simulink model "Simulator"  (R2015a)
settings: Solver=ode45  StartTime=0.0  StopTime=tsim  RelTol=1e-3
InitFcn:
  | Parameters
values from neighbouring files (symbols this model uses):
  delay_altitude = 1    [Parameters_controllers.m]
  delay_attitude = 1    [Parameters_controllers.m]
  delay_mixer = 1    [Parameters_controllers.m]
  dLMN = [dLdp  0   0 ... (first row only)    [Parameters.m]    (also in Parameters_quadrotor.m = [dL_dp  0    0)
  g = 9.81    [Parameters.m]
  In = diag([Ixx Iyy Izz])    [Parameters.m]
  InInv = In\eye(3)    [Parameters.m]
  K = param*sign    [Parameters.m]    (also in Parameters_controllers.m = [              -Kt,               -Kt,               -Kt,   )
  Kdp = 0.05    [Parameters.m]
  Kdq = 0.05    [Parameters.m]
  Kinv = K\eye(4)    [Parameters.m]    (also in Parameters_controllers.m = [ -1/(4*Kt),  2^(1/2)/(4*Kt*b),  2^(1/2)/(4*Kt*b), -1/(4*Kq))
  Kip = 0.3    [Parameters.m]
  Kiq = 0.3    [Parameters.m]
  Kir = 0.01    [Parameters.m]
  KPP = 1.1    [Parameters.m]
  Kpp = 0.3    [Parameters.m]
  Kpq = 0.3    [Parameters.m]
  Kpr = 0.08    [Parameters.m]
  KRP = 1.1    [Parameters.m]
  m = 1.5    [Parameters.m]
  Mb = diag([m m m])    [Parameters.m]
  MbInv = Mb\eye(3)    [Parameters.m]
  N = 1/Tf    (= 100)    [Parameters.m]
  pitchMax = pi/6    (= 0.523598775598)    [Parameters.m]
  rollMax = pi/6    (= 0.523598775598)    [Parameters.m]
  tau = 0.055257    [Parameters.m]
  x1 = [m q]    [Parameters.m]
undefined symbols (not defined in the file or in its folder): KaD, KaI, KaN, KaP, Kba, Kbp, Kbq, Kbr, KD, Kdr, KN, KP, KPD, KPI, KRD, KRI, KYD, KYP, magnitude, sat, sata, satp, satq, satr, sigbuilder_block, tc, U
libraries: simulink x9, aerolibutil x2
settings Model: Creator=pela  LastModifiedBy=Mattia
settings SolverCC: ZeroCrossAlgorithm=Adaptive
settings DataIOCC: LimitDataPoints=off

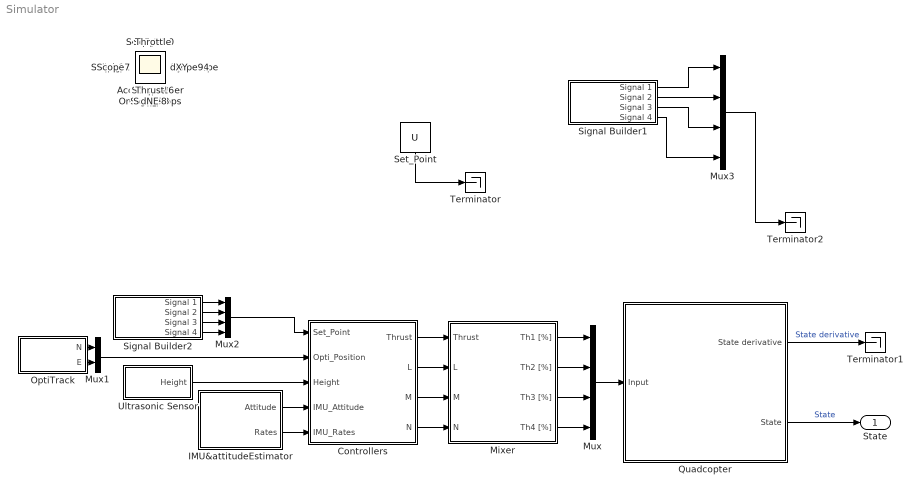
== system Simulator ==
  Controllers : Subsystem
  IMU&attitudeEstimator : Subsystem
  Mixer : Subsystem  InitFcn=|
      | %%Parameters definition
      | b = 0.55/2;
      | RPMmax = 3*4.2*710;
      | D = 12*2.54/100;
      | Ct = 0.001;
      | Cq = 0.001;
      | ro = 1.225;
      | 
      | %% From omega squared to forces/torques
      |  A = ro*D^4*diag([Ct b/sqrt(2)*Ct b/sqrt(2)*Ct Cq*D]);
      |  B = [ 1  1  1 1;
      |          1 -1 -1 1;
      |         -1 -1  1 1;
      |         -1  1 -1 1];
      |  C = inv(A*B);       %TM = C * omegasq
  Mux : Mux
  Mux1 : Mux  Inputs=2
  Mux2 : Mux
  Mux3 : Mux
  OptiTrack : Subsystem
  Quadcopter : Subsystem
      mask Display:
      | image(imread('quad.png'))
      | port_label('input',1,'u')
      | port_label('output',1,'Xdot')
      | port_label('output',2,'X')
  Set_Point : Constant  Value=U
  Signal Builder1 : Subsystem  Tag=STV Subsys  LoadFcn=sigbuilder_block('load');  StartFcn=sigbuilder_block('start');  StopFcn=sigbuilder_block('stop');  ClipboardFcn=sigbuilder_block('clipboard');  mask(Sigbuilder block){}
      mask help: Simulink:masks:SigbuilderBlock_MD
      mask init:
      | if ~strcmp(get_param(bdroot(gcbh),'SimulationStatus'),'stopped') tuvar = sigbuilder_block('maskInit'); end
      settings: CopyFcn=sigbuilder_block('copy');  DeleteFcn=sigbuilder_block('delete');  ModelCloseFcn=sigbuilder_block('modelClose');  PreSaveFcn=sigbuilder_block('preSave');  PauseFcn=sigbuilder_block('pause');  ContinueFcn=sigbuilder_block('continue');  NameChangeFcn=sigbuilder_block('namechange');  OpenFcn=sigbuilder_block('open',[5.4 30 1141.2 522.6 ]);  CloseFcn=sigbuilder_block('close');
      mask Display: plot(0, 0, 100, 100,[2, 2, 32, 32, 2], [68, 8, 8, 68, 68],[32, 2], [38, 38], [32, 19, 2],[53, 60, 44], [32, 17, 17, 2],[16, 16, 31, 31]);txt = getActiveGroup(gcbh);text(2, 100, txt,'verticalAlignment', 'top');
  Signal Builder2 : Subsystem  Tag=STV Subsys  LoadFcn=sigbuilder_block('load');  StartFcn=sigbuilder_block('start');  StopFcn=sigbuilder_block('stop');  ClipboardFcn=sigbuilder_block('clipboard');  mask(Sigbuilder block){}
      mask help: Simulink:masks:SigbuilderBlock_MD
      mask init:
      | if ~strcmp(get_param(bdroot(gcbh),'SimulationStatus'),'stopped') tuvar = sigbuilder_block('maskInit'); end
      settings: CopyFcn=sigbuilder_block('copy');  DeleteFcn=sigbuilder_block('delete');  ModelCloseFcn=sigbuilder_block('modelClose');  PreSaveFcn=sigbuilder_block('preSave');  PauseFcn=sigbuilder_block('pause');  ContinueFcn=sigbuilder_block('continue');  NameChangeFcn=sigbuilder_block('namechange');  OpenFcn=sigbuilder_block('open',[5.4 30 1141.2 522.6 ]);  CloseFcn=sigbuilder_block('close');
      mask Display: plot(0, 0, 100, 100,[2, 2, 32, 32, 2], [68, 8, 8, 68, 68],[32, 2], [38, 38], [32, 19, 2],[53, 60, 44], [32, 17, 17, 2],[16, 16, 31, 31]);txt = getActiveGroup(gcbh);text(2, 100, txt,'verticalAlignment', 'top');
  Terminator : Terminator
  Terminator1 : Terminator
  Terminator2 : Terminator
  Ultrasonic Sensor : Subsystem
  State : Outport
  Accelerometer : Scope
      settings: ShowLegends=on  YMin=-10  YMax=10  SaveName=ScopeData9
  Fg : Scope
      settings: ShowLegends=on  YMin=-10  YMax=10  SaveName=ScopeData4
  Fprops : Scope
      settings: ShowLegends=on  YMin=-22.13861  YMax=2.45985  SaveName=ScopeData2
  Gyroscope : Scope
      settings: ShowLegends=on  YMin=-10  YMax=10  SaveName=ScopeData10
  Height : Scope
      settings: ShowLegends=on  TimeRange=10  YMin=-0.2  YMax=1.4  SaveName=ScopeData5
  Moments : Scope
      settings: YMin=-1.875  YMax=1.875  SaveName=ScopeData7
  Mprops : Scope
      settings: ShowLegends=on  YMin=-0.25293  YMax=0.32754  SaveName=ScopeData3
  Omega_props : Scope
      settings: ShowLegends=on  TimeRange=10  YMin=328.24586  YMax=550.97691
  Scope{,1..16} (17 alike) : Scope
      Scope settings: YMin=-1.28463  YMax=0.42301  SaveName=ScopeData8
      Scope1 settings: YMin=-10  YMax=10  SaveName=ScopeData11
      Scope10 settings: YMin=-10  YMax=10  SaveName=ScopeData17
      Scope11 settings: YMin=-10  YMax=10  SaveName=ScopeData18
      Scope12 settings: YMin=103280.52588  YMax=299110.73241  SaveName=ScopeData19
      Scope13 settings: YMin=-10  YMax=10  SaveName=ScopeData23
      Scope14 settings: YMin=-10  YMax=10  SaveName=ScopeData26
      Scope15 settings: YMin=-0.00000000000000007  YMax=0.00000000000000005  SaveName=ScopeData27
      Scope16 settings: YMin=-0.07851  YMax=0.5905  SaveName=ScopeData28
      Scope2 settings: YMin=-10  YMax=10  SaveName=ScopeData12
      Scope3 settings: YMin=-10  YMax=10  SaveName=ScopeData13
      Scope4 settings: YMin=-10  YMax=10  SaveName=ScopeData14
      Scope5 settings: YMin=-10  YMax=10  SaveName=ScopeData15
      Scope6 settings: YMin=-10  YMax=10  SaveName=ScopeData20
      Scope7 settings: YMin=-0.0134  YMax=0.02255  SaveName=ScopeData21
      Scope8 settings: YMin=-0.0504  YMax=0.30441  SaveName=ScopeData22
      Scope9 settings: YMin=-10  YMax=10  SaveName=ScopeData16
  Throttle : Scope
      settings: ShowLegends=on  YMin=-12.5  YMax=112.5
  Thrust : Scope
      settings: YMin=-20.52889  YMax=-13.37103  SaveName=ScopeData6
  dNE : Scope
      settings: ShowLegends=on  YMin=-0.125  YMax=1.125  SaveName=ScopeData24
  dXY : Scope
      settings: YMin=-0.125  YMax=1.125  SaveName=ScopeData25
  wires:
  Quadcopter/2(State) -> State/1  "State"
  Mux/1 -> Quadcopter/1(Input)
  Mixer/1(Th1 [%]) -> Mux/1
  Mixer/2(Th2 [%]) -> Mux/2
  Mixer/3(Th3 [%]) -> Mux/3
  Mixer/4(Th4 [%]) -> Mux/4
  Quadcopter/1(State derivative) -> Terminator1/1  "State derivative"
  Ultrasonic Sensor/1(Height) -> Controllers/3(Height)
  Controllers/1(Thrust) -> Mixer/1(Thrust)
  Controllers/2(L) -> Mixer/2(L)
  Controllers/3(M) -> Mixer/3(M)
  Controllers/4(N) -> Mixer/4(N)
  IMU&attitudeEstimator/1(Attitude) -> Controllers/4(IMU_Attitude)
  IMU&attitudeEstimator/2(Rates) -> Controllers/5(IMU_Rates)
  Mux1/1 -> Controllers/2(Opti_Position)
  Mux2/1 -> Controllers/1(Set_Point)
  Set_Point/1 -> Terminator/1
  Signal Builder2/2(Signal 2) -> Mux2/2
  Signal Builder2/3(Signal 3) -> Mux2/3
  Signal Builder2/4(Signal 4) -> Mux2/4
  OptiTrack/1(N) -> Mux1/1
  OptiTrack/2(E) -> Mux1/2
  Signal Builder2/1(Signal 1) -> Mux2/1
  Mux3/1 -> Terminator2/1
  Signal Builder1/2(Signal 2) -> Mux3/2
  Signal Builder1/3(Signal 3) -> Mux3/3
  Signal Builder1/4(Signal 4) -> Mux3/4
  Signal Builder1/1(Signal 1) -> Mux3/1

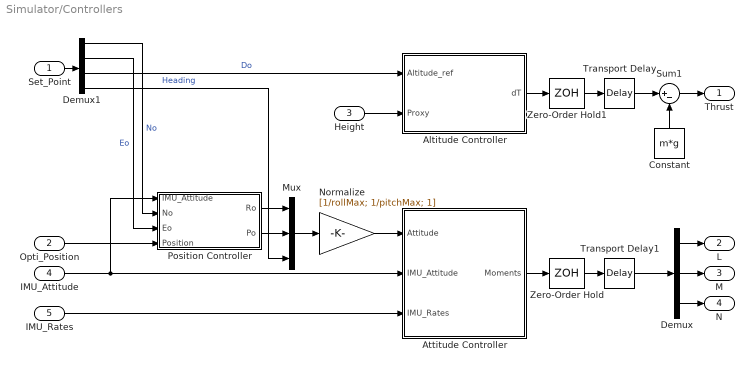
== system Simulator/Controllers ==
  Set_Point : Inport
  Opti_Position : Inport  Port=2
  Height : Inport  Port=3
  IMU_Attitude : Inport  Port=4
  IMU_Rates : Inport  Port=5
  Altitude Controller : Subsystem
  Attitude Controller : Subsystem
  Constant : Constant  Value=m*g
  Demux : Demux  Outputs=3
  Demux1 : Demux
  Mux : Mux  Inputs=3
  Normalize : Gain  Gain=[1/rollMax; 1/pitchMax; 1]
  Position Controller : Subsystem
  Sum1 : Sum  Inputs=|+-
  Transport Delay : TransportDelay  DelayTime=delay_altitude*tc
  Transport Delay1 : TransportDelay  DelayTime=delay_attitude*tc
  Zero-Order Hold : ZeroOrderHold  SampleTime=tc
  Zero-Order Hold1 : ZeroOrderHold  SampleTime=tc
  Thrust : Outport
  L : Outport  Port=2
  M : Outport  Port=3
  N : Outport  Port=4
  wires:
  Attitude Controller/1(Moments) -> Zero-Order Hold/1
  IMU_Rates/1 -> Attitude Controller/3(IMU_Rates)
  Demux/1 -> L/1
  Demux/2 -> M/1
  Demux/3 -> N/1
  Set_Point/1 -> Demux1/1
  IMU_Attitude/1 -> Position Controller/1(IMU_Attitude), Attitude Controller/2(IMU_Attitude)
  Mux/1 -> Normalize/1
  Normalize/1 -> Attitude Controller/1(Attitude)
  Sum1/1 -> Thrust/1
  Height/1 -> Altitude Controller/2(Proxy)
  Altitude Controller/1(dT) -> Zero-Order Hold1/1
  Zero-Order Hold/1 -> Transport Delay1/1
  Zero-Order Hold1/1 -> Transport Delay/1
  Transport Delay1/1 -> Demux/1
  Opti_Position/1 -> Position Controller/4(Position)
  Demux1/1 -> Position Controller/2(No)  "No"
  Demux1/2 -> Position Controller/3(Eo)  "Eo"
  Demux1/3 -> Altitude Controller/1(Altitude_ref)  "Do"
  Demux1/4 -> Mux/3  "Heading"
  Position Controller/1(Ro) -> Mux/1
  Position Controller/2(Po) -> Mux/2
  Transport Delay/1 -> Sum1/1
  Constant/1 -> Sum1/2

== system Simulator/IMU&attitudeEstimator ==
  Zero-Order Hold : ZeroOrderHold  SampleTime=tc
  Zero-Order Hold1 : ZeroOrderHold  SampleTime=tc
  Attitude : Outport
  Rates : Outport  Port=2
  wires:
  [Omega_b] -> Zero-Order Hold1/1
  [Alpha_e] -> Zero-Order Hold/1
  Zero-Order Hold/1 -> Attitude/1
  Zero-Order Hold1/1 -> Rates/1

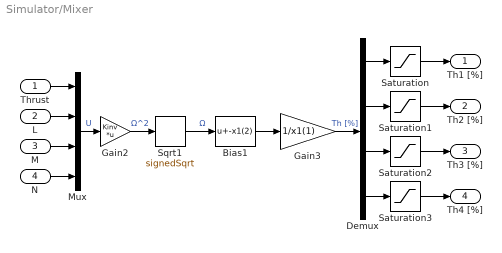
== system Simulator/Mixer ==
  Thrust : Inport
  L : Inport  Port=2
  M : Inport  Port=3
  N : Inport  Port=4
  Bias1 : Bias  Bias=-x1(2)
  Demux : Demux
  Gain2 : Gain  Gain=Kinv  Multiplication=Matrix(K*u)
  Gain3 : Gain  Gain=1/x1(1)
  Mux : Mux
  Saturation{,1..3} (4 alike) : Saturate  UpperLimit=100  LowerLimit=0
  Sqrt1 : Sqrt  Operator=signedSqrt  SaturateOnIntegerOverflow=on
  Th1 [%] : Outport
  Th2 [%] : Outport  Port=2
  Th3 [%] : Outport  Port=3
  Th4 [%] : Outport  Port=4
  wires:
  N/1 -> Mux/4
  M/1 -> Mux/3
  L/1 -> Mux/2
  Demux/1 -> Saturation/1
  Saturation/1 -> Th1 [%]/1
  Demux/2 -> Saturation1/1
  Demux/3 -> Saturation2/1
  Demux/4 -> Saturation3/1
  Saturation3/1 -> Th4 [%]/1
  Saturation2/1 -> Th3 [%]/1
  Saturation1/1 -> Th2 [%]/1
  Gain3/1 -> Demux/1  "Th [%]"
  Bias1/1 -> Gain3/1
  Gain2/1 -> Sqrt1/1  "Ω^2"
  Mux/1 -> Gain2/1  "U"
  Sqrt1/1 -> Bias1/1  "Ω"
  Thrust/1 -> Mux/1

== system Simulator/OptiTrack ==
  Demux : Demux  Outputs=3
  Terminator : Terminator
  N : Outport
  E : Outport  Port=2
  wires:
  Demux/1 -> N/1  "N"
  Demux/3 -> Terminator/1  "D"
  [P_e] -> Demux/1
  Demux/2 -> E/1  "E"

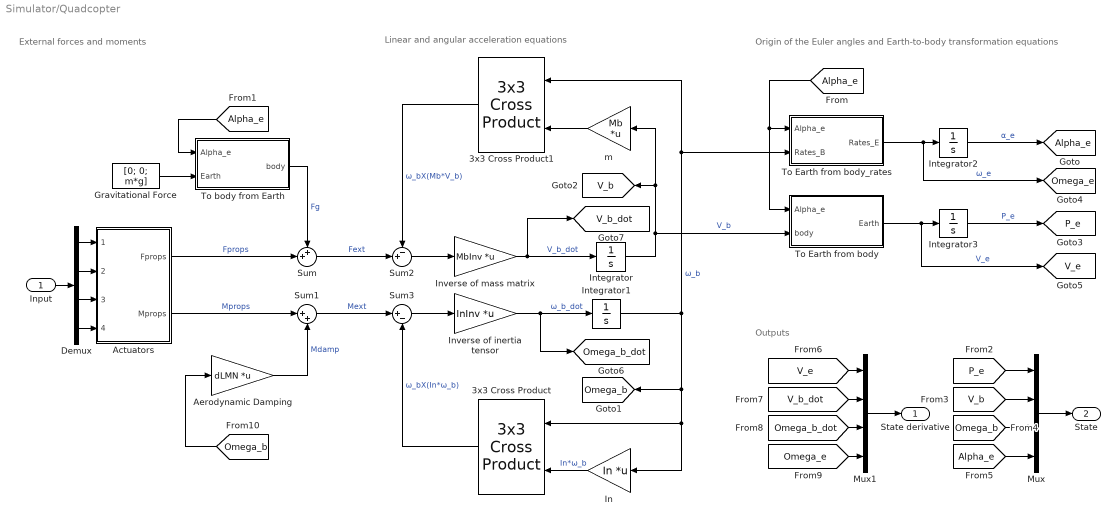
== system Simulator/Quadcopter ==
  note: External forces and moments
  note: Outputs
  note: Origin of the Euler angles and Earth-to-body transformation equations
  note: Linear and angular acceleration equations
  Input : Inport
  3x3 Cross Product : aerolibutil/3x3 Cross Product
  3x3 Cross Product1 : aerolibutil/3x3 Cross Product
  Actuators : Subsystem
  Aerodynamic Damping : Gain  Gain=dLMN  Multiplication=Matrix(K*u)
  Demux : Demux
  Gravitational Force : Constant  Value=[0; 0; m*g]
  In : Gain  Gain=In  Multiplication=Matrix(K*u)
  Integrator{,1..3} (4 alike) : Integrator  InitialCondition=[0; 0; 0]
  Inverse of inertia tensor : Gain  Gain=InInv  Multiplication=Matrix(K*u)
  Inverse of mass matrix : Gain  Gain=MbInv  Multiplication=Matrix(K*u)
  Mux : Mux
  Mux1 : Mux
  Sum : Sum  Inputs=++|
  Sum1 : Sum  Inputs=|++
  Sum2 : Sum  Inputs=-+|
  Sum3 : Sum  Inputs=|+-
  To Earth from body : MATLAB Function  TreatAsAtomicUnit=on
  To Earth from body_rates : MATLAB Function  TreatAsAtomicUnit=on
  To body from Earth : MATLAB Function  TreatAsAtomicUnit=on
  m : Gain  Gain=Mb  Multiplication=Matrix(K*u)
  State derivative : Outport
  State : Outport  Port=2
  tag scope: Alpha_e=global, Omega_b=global, Omega_b_dot=global, Omega_e=global, P_e=global, V_b=global, V_b_dot=global, V_e=global
  wires:
  To Earth from body_rates/1(Rates_E) -> Integrator2/1, [Omega_e]  "ω_e"
  [P_e] -> Mux/1
  Actuators/2(Mprops) -> Sum1/1  "Mprops"
  Input/1 -> Demux/1
  3x3 Cross Product/1 -> Sum3/2  "ω_bX(In*ω_b)"
  [V_b_dot] -> Mux1/2
  Mux/1 -> State/1
  Mux1/1 -> State derivative/1
  [V_b] -> Mux/2
  [Alpha_e] -> Mux/4
  [Omega_b] -> Mux/3
  Demux/4 -> Actuators/4(Th4 [%])
  [Omega_e] -> Mux1/4
  [Omega_b_dot] -> Mux1/3
  [V_e] -> Mux1/1
  Demux/3 -> Actuators/3(Th3 [%])
  Inverse of mass matrix/1 -> Integrator/1, [V_b_dot]  "V_b_dot"
  Integrator/1 -> To Earth from body/2(body), m/1, [V_b]  "V_b"
  [Alpha_e] -> To Earth from body/1(Alpha_e), To Earth from body_rates/1(Alpha_e)
  Integrator1/1 -> To Earth from body_rates/2(Rates_B), 3x3 Cross Product1/1, 3x3 Cross Product/1, In/1, [Omega_b]  "ω_b"
  Sum3/1 -> Inverse of inertia tensor/1
  Sum2/1 -> Inverse of mass matrix/1
  m/1 -> 3x3 Cross Product1/2
  Sum/1 -> Sum2/2  "Fext"
  Sum1/1 -> Sum3/1  "Mext"
  Demux/1 -> Actuators/1(Th1 [%])
  Demux/2 -> Actuators/2(Th2 [%])
  Inverse of inertia tensor/1 -> Integrator1/1, [Omega_b_dot]  "ω_b_dot"
  3x3 Cross Product1/1 -> Sum2/1  "ω_bX(Mb*V_b)"
  Integrator2/1 -> [Alpha_e]  "α_e"
  Aerodynamic Damping/1 -> Sum1/2  "Mdamp"
  Actuators/1(Fprops) -> Sum/2  "Fprops"
  Integrator3/1 -> [P_e]  "P_e"
  In/1 -> 3x3 Cross Product/2  "In*ω_b"
  [Omega_b] -> Aerodynamic Damping/1
  To Earth from body/1(Earth) -> [V_e], Integrator3/1  "V_e"
  To body from Earth/1(body) -> Sum/1  "Fg"
  Gravitational Force/1 -> To body from Earth/2(Earth)
  [Alpha_e] -> To body from Earth/1(Alpha_e)

== system Simulator/Signal Builder1 ==
  Demux : Demux  Tag=STV Demux
  FromWs : FromWorkspace  Tag=STV FromWs  VariableName=tuvar  SampleTime=0
      SigBuilderData=|
      | common.afterFinalStr = 'Extrapolate'
      | common.sampleTime = 0
      | dataSet.timeRange = [0 50]
      | dataSet.name = 'Group 1'
      | sbobj.Groups.Name = 'Group 1'
      | sbobj.Groups.Signals(1).Name = 'Signal 1'
      | sbobj.Groups.Signals(1).XData = [0 25 25 35 35 50]
      | sbobj.Groups.Signals(1).YData = [0 0 1 1 0 0]
      | sbobj.Groups.Signals(2).Name = 'Signal 2'
      | sbobj.Groups.Signals(2).XData = [0 15 15 30 30 50]
      | sbobj.Groups.Signals(2).YData = [0 0 1 1 0 0]
      | sbobj.Groups.Signals(3).Name = 'Signal 3'
      | sbobj.Groups.Signals(3).XData = [0 5 40 45 50]
      | sbobj.Groups.Signals(3).YData = [0 -1 -1 0 0]
      | sbobj.Groups.Signals(4).Name = 'Signal 4'
      | sbobj.Groups.Signals(4).XData = [0 10 10 20 20 50]
      | sbobj.Groups.Signals(4).YData = [0 0 1.57079632679 1.57079632679 0 0]
      | sbobj.Groups.TimeRange = [0 50]
  Signal 1 : Outport  Tag=STV Outport
  Signal 2 : Outport  Tag=STV Outport  Port=2
  Signal 3 : Outport  Tag=STV Outport  Port=3
  Signal 4 : Outport  Tag=STV Outport  Port=4
  wires:
  Demux/4 -> Signal 4/1
  Demux/3 -> Signal 3/1
  Demux/2 -> Signal 2/1
  Demux/1 -> Signal 1/1
  FromWs/1 -> Demux/1

== system Simulator/Signal Builder2 ==
  Demux : Demux  Tag=STV Demux
  FromWs : FromWorkspace  Tag=STV FromWs  VariableName=tuvar  SampleTime=0
      SigBuilderData=|
      | common.afterFinalStr = 'Extrapolate'
      | common.sampleTime = 0
      | dataSet.timeRange = [0 50]
      | dataSet.name = 'Group 1'
      | sbobj.Groups.Name = 'Group 1'
      | sbobj.Groups.Signals(1).Name = 'Signal 1'
      | sbobj.Groups.Signals(1).XData = [0 20 20 30 30 50]
      | sbobj.Groups.Signals(1).YData = [0 0 1 1 0 0]
      | sbobj.Groups.Signals(2).Name = 'Signal 2'
      | sbobj.Groups.Signals(2).XData = [0 15 15 25 25 50]
      | sbobj.Groups.Signals(2).YData = [0 0 1 1 0 0]
      | sbobj.Groups.Signals(3).Name = 'Signal 3'
      | sbobj.Groups.Signals(3).XData = [0 5 40 45 50]
      | sbobj.Groups.Signals(3).YData = [0 -1 -1 0 0]
      | sbobj.Groups.Signals(4).Name = 'Signal 4'
      | sbobj.Groups.Signals(4).XData = [0 50]
      | sbobj.Groups.Signals(4).YData = [0 0]
      | sbobj.Groups.TimeRange = [0 50]
  Signal 1 : Outport  Tag=STV Outport
  Signal 2 : Outport  Tag=STV Outport  Port=2
  Signal 3 : Outport  Tag=STV Outport  Port=3
  Signal 4 : Outport  Tag=STV Outport  Port=4
  wires:
  FromWs/1 -> Demux/1
  Demux/1 -> Signal 1/1
  Demux/2 -> Signal 2/1
  Demux/3 -> Signal 3/1
  Demux/4 -> Signal 4/1

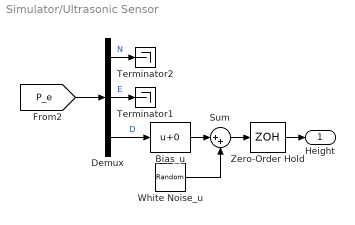
== system Simulator/Ultrasonic Sensor ==
  Bias_u : Bias
  Demux : Demux  Outputs=3
  Sum : Sum  Inputs=|++
  Terminator1 : Terminator
  Terminator2 : Terminator
  White Noise_u : RandomNumber  DisableCoverage=on  Variance=0*0.00001  SampleTime=0.01
  Zero-Order Hold : ZeroOrderHold  SampleTime=tc
  Height : Outport
  wires:
  Sum/1 -> Zero-Order Hold/1
  Demux/2 -> Terminator1/1  "E"
  [P_e] -> Demux/1
  Bias_u/1 -> Sum/1
  White Noise_u/1 -> Sum/2
  Demux/1 -> Terminator2/1  "N"
  Zero-Order Hold/1 -> Height/1
  Demux/3 -> Bias_u/1  "D"

== system Simulator/Controllers/Altitude Controller ==
  note: Altitude Controller
  Altitude_ref : Inport
  Proxy : Inport  Port=2
  PID Controller : simulink/Continuous/PID Controller  Controller=PID  TimeDomain=Continuous-time  SampleTime=-1  IntegratorMethod=Forward Euler  FilterMethod=Trapezoidal  Form=Parallel  UseFilter=on  ControllerParametersSource=internal  P=KaP  I=KaI  D=KaD  N=KaN  InitialConditionSource=internal  InitialConditionForIntegrator=0  InitialConditionForFilter=0  ExternalReset=none  LimitOutput=on  UpperSaturationLimit=sata  LowerSaturationLimit=-sata  LinearizeAsGain=on  AntiWindupMode=back-calculation  Kb=Kba  TrackingMode=off  Kt=1  PParamMin=[]  PParamMax=[]  IParamMin=[]  IParamMax=[]  DParamMin=[]  DParamMax=[]  NParamMin=[]  NParamMax=[]  KbParamMin=[]  KbParamMax=[]  KtParamMin=[]  KtParamMax=[]  POutMin=[]  POutMax=[]  IOutMin=[]  IOutMax=[]  DOutMin=[]  DOutMax=[]  NOutMin=[]  NOutMax=[]  KbOutMin=[]  KbOutMax=[]  KtOutMin=[]  KtOutMax=[]  IntegratorOutMin=[]  IntegratorOutMax=[]  FilterOutMin=[]  FilterOutMax=[]  SumOutMin=[]  SumOutMax=[]  SumI1OutMin=[]  SumI1OutMax=[]  SumI2OutMin=[]  SumI2OutMax=[]  SumI3OutMin=[]  SumI3OutMax=[]  SumDOutMin=[]  SumDOutMax=[]  SaturationOutMin=[]  SaturationOutMax=[]  IntegratorContinuousStateAttributes=''  IntegratorStateMustResolveToSignalObject=off  IntegratorRTWStateStorageClass=Auto  FilterContinuousStateAttributes=''  FilterStateMustResolveToSignalObject=off  FilterRTWStateStorageClass=Auto  DifferentiatorICPrevScaledInput=0  DifferentiatorOutMin=[]  DifferentiatorOutMax=[]
  Sum2 : Sum  Inputs=|+-
  dT : Outport
  wires:
  Sum2/1 -> PID Controller/1
  Altitude_ref/1 -> Sum2/1
  Proxy/1 -> Sum2/2
  PID Controller/1 -> dT/1

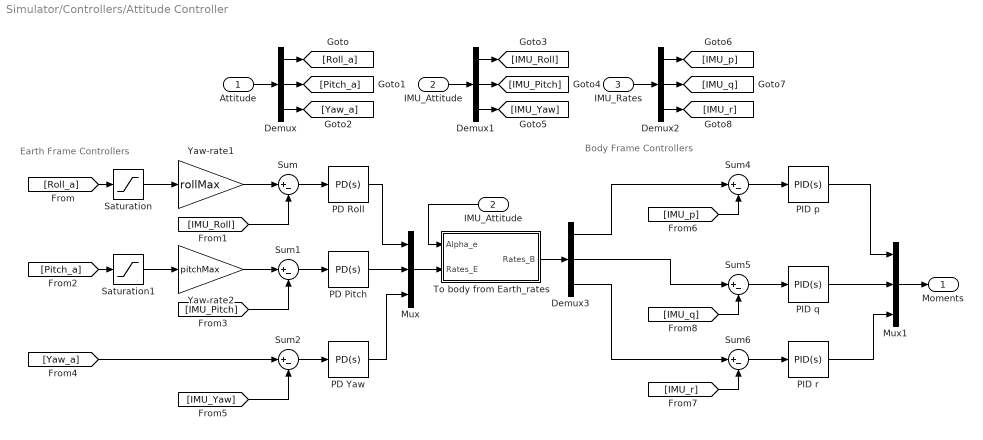
== system Simulator/Controllers/Attitude Controller ==
  note: Body Frame Controllers
  note: Earth Frame Controllers
  Attitude : Inport
  IMU_Attitude : Inport  Port=2
  IMU_Rates : Inport  Port=3
  Demux{,1..3} (4 alike) : Demux  Outputs=3
  "IMU_Attitude " : InportShadow  Port=2
  Mux : Mux  Inputs=3
  Mux1 : Mux  Inputs=3
  PD Pitch : simulink/Continuous/PID Controller  Controller=PD  TimeDomain=Continuous-time  SampleTime=-1  IntegratorMethod=Forward Euler  FilterMethod=Forward Euler  Form=Parallel  UseFilter=on  ControllerParametersSource=internal  P=KPP  I=KPI  D=KPD  N=N  InitialConditionSource=internal  InitialConditionForIntegrator=0  InitialConditionForFilter=0  ExternalReset=none  LimitOutput=off  UpperSaturationLimit=inf  LowerSaturationLimit=-inf  LinearizeAsGain=on  AntiWindupMode=none  Kb=1  TrackingMode=off  Kt=1  PParamMin=[]  PParamMax=[]  IParamMin=[]  IParamMax=[]  DParamMin=[]  DParamMax=[]  NParamMin=[]  NParamMax=[]  KbParamMin=[]  KbParamMax=[]  KtParamMin=[]  KtParamMax=[]  POutMin=[]  POutMax=[]  IOutMin=[]  IOutMax=[]  DOutMin=[]  DOutMax=[]  NOutMin=[]  NOutMax=[]  KbOutMin=[]  KbOutMax=[]  KtOutMin=[]  KtOutMax=[]  IntegratorOutMin=[]  IntegratorOutMax=[]  FilterOutMin=[]  FilterOutMax=[]  SumOutMin=[]  SumOutMax=[]  SumI1OutMin=[]  SumI1OutMax=[]  SumI2OutMin=[]  SumI2OutMax=[]  SumI3OutMin=[]  SumI3OutMax=[]  SumDOutMin=[]  SumDOutMax=[]  SaturationOutMin=[]  SaturationOutMax=[]  IntegratorContinuousStateAttributes=''  IntegratorStateMustResolveToSignalObject=off  IntegratorRTWStateStorageClass=Auto  FilterContinuousStateAttributes=''  FilterStateMustResolveToSignalObject=off  FilterRTWStateStorageClass=Auto  DifferentiatorICPrevScaledInput=0  DifferentiatorOutMin=[]  DifferentiatorOutMax=[]
  PD Roll : simulink/Continuous/PID Controller  Controller=PD  TimeDomain=Continuous-time  SampleTime=-1  IntegratorMethod=Forward Euler  FilterMethod=Forward Euler  Form=Parallel  UseFilter=on  ControllerParametersSource=internal  P=KRP  I=KRI  D=KRD  N=N  InitialConditionSource=internal  InitialConditionForIntegrator=0  InitialConditionForFilter=0  ExternalReset=none  LimitOutput=off  UpperSaturationLimit=inf  LowerSaturationLimit=-inf  LinearizeAsGain=on  AntiWindupMode=none  Kb=1  TrackingMode=off  Kt=1  PParamMin=[]  PParamMax=[]  IParamMin=[]  IParamMax=[]  DParamMin=[]  DParamMax=[]  NParamMin=[]  NParamMax=[]  KbParamMin=[]  KbParamMax=[]  KtParamMin=[]  KtParamMax=[]  POutMin=[]  POutMax=[]  IOutMin=[]  IOutMax=[]  DOutMin=[]  DOutMax=[]  NOutMin=[]  NOutMax=[]  KbOutMin=[]  KbOutMax=[]  KtOutMin=[]  KtOutMax=[]  IntegratorOutMin=[]  IntegratorOutMax=[]  FilterOutMin=[]  FilterOutMax=[]  SumOutMin=[]  SumOutMax=[]  SumI1OutMin=[]  SumI1OutMax=[]  SumI2OutMin=[]  SumI2OutMax=[]  SumI3OutMin=[]  SumI3OutMax=[]  SumDOutMin=[]  SumDOutMax=[]  SaturationOutMin=[]  SaturationOutMax=[]  IntegratorContinuousStateAttributes=''  IntegratorStateMustResolveToSignalObject=off  IntegratorRTWStateStorageClass=Auto  FilterContinuousStateAttributes=''  FilterStateMustResolveToSignalObject=off  FilterRTWStateStorageClass=Auto  DifferentiatorICPrevScaledInput=0  DifferentiatorOutMin=[]  DifferentiatorOutMax=[]
  PD Yaw : simulink/Continuous/PID Controller  Controller=PD  TimeDomain=Continuous-time  SampleTime=-1  IntegratorMethod=Forward Euler  FilterMethod=Forward Euler  Form=Parallel  UseFilter=on  ControllerParametersSource=internal  P=KYP  I=KPI  D=KYD  N=N  InitialConditionSource=internal  InitialConditionForIntegrator=0  InitialConditionForFilter=0  ExternalReset=none  LimitOutput=off  UpperSaturationLimit=inf  LowerSaturationLimit=-inf  LinearizeAsGain=on  AntiWindupMode=none  Kb=1  TrackingMode=off  Kt=1  PParamMin=[]  PParamMax=[]  IParamMin=[]  IParamMax=[]  DParamMin=[]  DParamMax=[]  NParamMin=[]  NParamMax=[]  KbParamMin=[]  KbParamMax=[]  KtParamMin=[]  KtParamMax=[]  POutMin=[]  POutMax=[]  IOutMin=[]  IOutMax=[]  DOutMin=[]  DOutMax=[]  NOutMin=[]  NOutMax=[]  KbOutMin=[]  KbOutMax=[]  KtOutMin=[]  KtOutMax=[]  IntegratorOutMin=[]  IntegratorOutMax=[]  FilterOutMin=[]  FilterOutMax=[]  SumOutMin=[]  SumOutMax=[]  SumI1OutMin=[]  SumI1OutMax=[]  SumI2OutMin=[]  SumI2OutMax=[]  SumI3OutMin=[]  SumI3OutMax=[]  SumDOutMin=[]  SumDOutMax=[]  SaturationOutMin=[]  SaturationOutMax=[]  IntegratorContinuousStateAttributes=''  IntegratorStateMustResolveToSignalObject=off  IntegratorRTWStateStorageClass=Auto  FilterContinuousStateAttributes=''  FilterStateMustResolveToSignalObject=off  FilterRTWStateStorageClass=Auto  DifferentiatorICPrevScaledInput=0  DifferentiatorOutMin=[]  DifferentiatorOutMax=[]
  PID p : simulink/Continuous/PID Controller  Controller=PID  TimeDomain=Continuous-time  SampleTime=-1  IntegratorMethod=Forward Euler  FilterMethod=Forward Euler  Form=Parallel  UseFilter=on  ControllerParametersSource=internal  P=Kpp  I=Kip  D=Kdp  N=N  InitialConditionSource=internal  InitialConditionForIntegrator=0  InitialConditionForFilter=0  ExternalReset=none  LimitOutput=on  UpperSaturationLimit=satp  LowerSaturationLimit=-satp  LinearizeAsGain=on  AntiWindupMode=back-calculation  Kb=Kbp  TrackingMode=off  Kt=1  PParamMin=[]  PParamMax=[]  IParamMin=[]  IParamMax=[]  DParamMin=[]  DParamMax=[]  NParamMin=[]  NParamMax=[]  KbParamMin=[]  KbParamMax=[]  KtParamMin=[]  KtParamMax=[]  POutMin=[]  POutMax=[]  IOutMin=[]  IOutMax=[]  DOutMin=[]  DOutMax=[]  NOutMin=[]  NOutMax=[]  KbOutMin=[]  KbOutMax=[]  KtOutMin=[]  KtOutMax=[]  IntegratorOutMin=[]  IntegratorOutMax=[]  FilterOutMin=[]  FilterOutMax=[]  SumOutMin=[]  SumOutMax=[]  SumI1OutMin=[]  SumI1OutMax=[]  SumI2OutMin=[]  SumI2OutMax=[]  SumI3OutMin=[]  SumI3OutMax=[]  SumDOutMin=[]  SumDOutMax=[]  SaturationOutMin=[]  SaturationOutMax=[]  IntegratorContinuousStateAttributes=''  IntegratorStateMustResolveToSignalObject=off  IntegratorRTWStateStorageClass=Auto  FilterContinuousStateAttributes=''  FilterStateMustResolveToSignalObject=off  FilterRTWStateStorageClass=Auto  DifferentiatorICPrevScaledInput=0  DifferentiatorOutMin=[]  DifferentiatorOutMax=[]
  PID q : simulink/Continuous/PID Controller  Controller=PID  TimeDomain=Continuous-time  SampleTime=-1  IntegratorMethod=Forward Euler  FilterMethod=Forward Euler  Form=Parallel  UseFilter=on  ControllerParametersSource=internal  P=Kpq  I=Kiq  D=Kdq  N=N  InitialConditionSource=internal  InitialConditionForIntegrator=0  InitialConditionForFilter=0  ExternalReset=none  LimitOutput=on  UpperSaturationLimit=satq  LowerSaturationLimit=-satq  LinearizeAsGain=on  AntiWindupMode=back-calculation  Kb=Kbq  TrackingMode=off  Kt=1  PParamMin=[]  PParamMax=[]  IParamMin=[]  IParamMax=[]  DParamMin=[]  DParamMax=[]  NParamMin=[]  NParamMax=[]  KbParamMin=[]  KbParamMax=[]  KtParamMin=[]  KtParamMax=[]  POutMin=[]  POutMax=[]  IOutMin=[]  IOutMax=[]  DOutMin=[]  DOutMax=[]  NOutMin=[]  NOutMax=[]  KbOutMin=[]  KbOutMax=[]  KtOutMin=[]  KtOutMax=[]  IntegratorOutMin=[]  IntegratorOutMax=[]  FilterOutMin=[]  FilterOutMax=[]  SumOutMin=[]  SumOutMax=[]  SumI1OutMin=[]  SumI1OutMax=[]  SumI2OutMin=[]  SumI2OutMax=[]  SumI3OutMin=[]  SumI3OutMax=[]  SumDOutMin=[]  SumDOutMax=[]  SaturationOutMin=[]  SaturationOutMax=[]  IntegratorContinuousStateAttributes=''  IntegratorStateMustResolveToSignalObject=off  IntegratorRTWStateStorageClass=Auto  FilterContinuousStateAttributes=''  FilterStateMustResolveToSignalObject=off  FilterRTWStateStorageClass=Auto  DifferentiatorICPrevScaledInput=0  DifferentiatorOutMin=[]  DifferentiatorOutMax=[]
  PID r : simulink/Continuous/PID Controller  Controller=PID  TimeDomain=Continuous-time  SampleTime=-1  IntegratorMethod=Forward Euler  FilterMethod=Forward Euler  Form=Parallel  UseFilter=on  ControllerParametersSource=internal  P=Kpr  I=Kir  D=Kdr  N=N  InitialConditionSource=internal  InitialConditionForIntegrator=0  InitialConditionForFilter=0  ExternalReset=none  LimitOutput=on  UpperSaturationLimit=satr  LowerSaturationLimit=-satr  LinearizeAsGain=on  AntiWindupMode=back-calculation  Kb=Kbr  TrackingMode=off  Kt=1  PParamMin=[]  PParamMax=[]  IParamMin=[]  IParamMax=[]  DParamMin=[]  DParamMax=[]  NParamMin=[]  NParamMax=[]  KbParamMin=[]  KbParamMax=[]  KtParamMin=[]  KtParamMax=[]  POutMin=[]  POutMax=[]  IOutMin=[]  IOutMax=[]  DOutMin=[]  DOutMax=[]  NOutMin=[]  NOutMax=[]  KbOutMin=[]  KbOutMax=[]  KtOutMin=[]  KtOutMax=[]  IntegratorOutMin=[]  IntegratorOutMax=[]  FilterOutMin=[]  FilterOutMax=[]  SumOutMin=[]  SumOutMax=[]  SumI1OutMin=[]  SumI1OutMax=[]  SumI2OutMin=[]  SumI2OutMax=[]  SumI3OutMin=[]  SumI3OutMax=[]  SumDOutMin=[]  SumDOutMax=[]  SaturationOutMin=[]  SaturationOutMax=[]  IntegratorContinuousStateAttributes=''  IntegratorStateMustResolveToSignalObject=off  IntegratorRTWStateStorageClass=Auto  FilterContinuousStateAttributes=''  FilterStateMustResolveToSignalObject=off  FilterRTWStateStorageClass=Auto  DifferentiatorICPrevScaledInput=0  DifferentiatorOutMin=[]  DifferentiatorOutMax=[]
  Saturation : Saturate  UpperLimit=1  LowerLimit=-1
  Saturation1 : Saturate  UpperLimit=1  LowerLimit=-1
  Sum{,1..2,4..6} (6 alike) : Sum  Inputs=|+-
  To body from Earth_rates : MATLAB Function  TreatAsAtomicUnit=on
  Yaw-rate1 : Gain  Gain=rollMax
  Yaw-rate2 : Gain  Gain=pitchMax
  Moments : Outport
  wires:
  Sum4/1 -> PID p/1
  IMU_Attitude/1 -> Demux1/1
  Attitude/1 -> Demux/1
  Demux/3 -> [Yaw_a]
  IMU_Rates/1 -> Demux2/1
  [IMU_Pitch] -> Sum1/2
  [Pitch_a] -> Saturation1/1
  [IMU_Roll] -> Sum/2
  [Roll_a] -> Saturation/1
  Mux1/1 -> Moments/1
  PD Roll/1 -> Mux/1
  Sum5/1 -> PID q/1
  PID r/1 -> Mux1/3
  PID p/1 -> Mux1/1
  Sum6/1 -> PID r/1
  PID q/1 -> Mux1/2
  Demux/2 -> [Pitch_a]
  Demux2/3 -> [IMU_r]
  Demux1/1 -> [IMU_Roll]
  Demux/1 -> [Roll_a]
  Demux2/1 -> [IMU_p]
  Demux1/3 -> [IMU_Yaw]
  Demux2/2 -> [IMU_q]
  Demux1/2 -> [IMU_Pitch]
  Sum/1 -> PD Roll/1
  Sum1/1 -> PD Pitch/1
  "IMU_Attitude "/1 -> To body from Earth_rates/1(Alpha_e)
  To body from Earth_rates/1(Rates_B) -> Demux3/1
  Mux/1 -> To body from Earth_rates/2(Rates_E)
  Yaw-rate1/1 -> Sum/1
  Yaw-rate2/1 -> Sum1/1
  Demux3/1 -> Sum4/1
  [IMU_p] -> Sum4/2
  Demux3/3 -> Sum6/1
  [IMU_q] -> Sum5/2
  [IMU_r] -> Sum6/2
  PD Pitch/1 -> Mux/2
  Demux3/2 -> Sum5/1
  Saturation/1 -> Yaw-rate1/1
  Saturation1/1 -> Yaw-rate2/1
  [IMU_Yaw] -> Sum2/2
  Sum2/1 -> PD Yaw/1
  [Yaw_a] -> Sum2/1
  PD Yaw/1 -> Mux/3

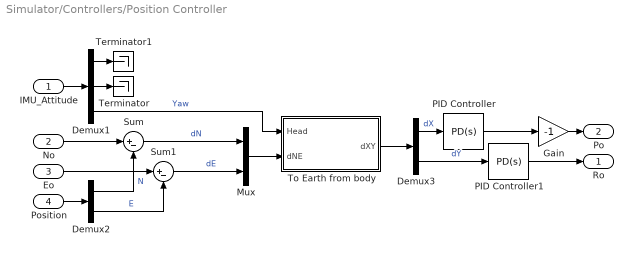
== system Simulator/Controllers/Position Controller ==
  IMU_Attitude : Inport
  No : Inport  Port=2
  Eo : Inport  Port=3
  Position : Inport  Port=4
  Demux1 : Demux  Outputs=3
  Demux2 : Demux  Outputs=2
  Demux3 : Demux  Outputs=2
  Gain : Gain  Gain=-1
  Mux : Mux  Inputs=2
  PID Controller : simulink/Continuous/PID Controller  Controller=PD  TimeDomain=Continuous-time  SampleTime=-1  IntegratorMethod=Forward Euler  FilterMethod=Forward Euler  Form=Parallel  UseFilter=on  ControllerParametersSource=internal  P=KP  I=0.01  D=KD  N=KN  InitialConditionSource=internal  InitialConditionForIntegrator=0  InitialConditionForFilter=0  ExternalReset=none  LimitOutput=on  UpperSaturationLimit=sat  LowerSaturationLimit=-sat  LinearizeAsGain=on  AntiWindupMode=none  Kb=1  TrackingMode=off  Kt=1  PParamMin=[]  PParamMax=[]  IParamMin=[]  IParamMax=[]  DParamMin=[]  DParamMax=[]  NParamMin=[]  NParamMax=[]  KbParamMin=[]  KbParamMax=[]  KtParamMin=[]  KtParamMax=[]  POutMin=[]  POutMax=[]  IOutMin=[]  IOutMax=[]  DOutMin=[]  DOutMax=[]  NOutMin=[]  NOutMax=[]  KbOutMin=[]  KbOutMax=[]  KtOutMin=[]  KtOutMax=[]  IntegratorOutMin=[]  IntegratorOutMax=[]  FilterOutMin=[]  FilterOutMax=[]  SumOutMin=[]  SumOutMax=[]  SumI1OutMin=[]  SumI1OutMax=[]  SumI2OutMin=[]  SumI2OutMax=[]  SumI3OutMin=[]  SumI3OutMax=[]  SumDOutMin=[]  SumDOutMax=[]  SaturationOutMin=[]  SaturationOutMax=[]  IntegratorContinuousStateAttributes=''  IntegratorStateMustResolveToSignalObject=off  IntegratorRTWStateStorageClass=Auto  FilterContinuousStateAttributes=''  FilterStateMustResolveToSignalObject=off  FilterRTWStateStorageClass=Auto  DifferentiatorICPrevScaledInput=0  DifferentiatorOutMin=[]  DifferentiatorOutMax=[]
  PID Controller1 : simulink/Continuous/PID Controller  Controller=PD  TimeDomain=Continuous-time  SampleTime=-1  IntegratorMethod=Forward Euler  FilterMethod=Forward Euler  Form=Parallel  UseFilter=on  ControllerParametersSource=internal  P=KP  I=0.01  D=KD  N=KN  InitialConditionSource=internal  InitialConditionForIntegrator=0  InitialConditionForFilter=0  ExternalReset=none  LimitOutput=on  UpperSaturationLimit=sat  LowerSaturationLimit=-sat  LinearizeAsGain=on  AntiWindupMode=none  Kb=1  TrackingMode=off  Kt=1  PParamMin=[]  PParamMax=[]  IParamMin=[]  IParamMax=[]  DParamMin=[]  DParamMax=[]  NParamMin=[]  NParamMax=[]  KbParamMin=[]  KbParamMax=[]  KtParamMin=[]  KtParamMax=[]  POutMin=[]  POutMax=[]  IOutMin=[]  IOutMax=[]  DOutMin=[]  DOutMax=[]  NOutMin=[]  NOutMax=[]  KbOutMin=[]  KbOutMax=[]  KtOutMin=[]  KtOutMax=[]  IntegratorOutMin=[]  IntegratorOutMax=[]  FilterOutMin=[]  FilterOutMax=[]  SumOutMin=[]  SumOutMax=[]  SumI1OutMin=[]  SumI1OutMax=[]  SumI2OutMin=[]  SumI2OutMax=[]  SumI3OutMin=[]  SumI3OutMax=[]  SumDOutMin=[]  SumDOutMax=[]  SaturationOutMin=[]  SaturationOutMax=[]  IntegratorContinuousStateAttributes=''  IntegratorStateMustResolveToSignalObject=off  IntegratorRTWStateStorageClass=Auto  FilterContinuousStateAttributes=''  FilterStateMustResolveToSignalObject=off  FilterRTWStateStorageClass=Auto  DifferentiatorICPrevScaledInput=0  DifferentiatorOutMin=[]  DifferentiatorOutMax=[]
  Sum : Sum  Inputs=|+-
  Sum1 : Sum  Inputs=|+-
  Terminator : Terminator
  Terminator1 : Terminator
  To Earth from body : MATLAB Function  TreatAsAtomicUnit=on
  Ro : Outport
  Po : Outport  Port=2
  wires:
  IMU_Attitude/1 -> Demux1/1
  Demux1/1 -> Terminator1/1
  Demux1/3 -> To Earth from body/1(Head)  "Yaw"
  Demux1/2 -> Terminator/1
  Position/1 -> Demux2/1
  No/1 -> Sum/1
  Demux2/1 -> Sum/2  "N"
  Eo/1 -> Sum1/1
  Demux2/2 -> Sum1/2  "E"
  Sum/1 -> Mux/1  "dN"
  Sum1/1 -> Mux/2  "dE"
  Mux/1 -> To Earth from body/2(dNE)
  To Earth from body/1(dXY) -> Demux3/1
  Demux3/2 -> PID Controller1/1  "dY"
  Demux3/1 -> PID Controller/1  "dX"
  PID Controller1/1 -> Ro/1
  PID Controller/1 -> Gain/1
  Gain/1 -> Po/1

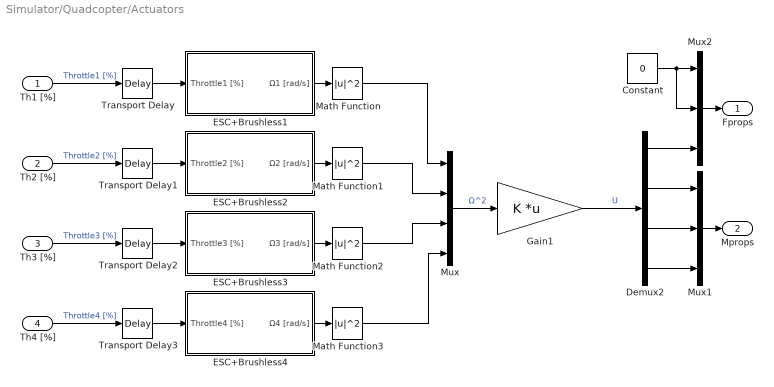
== system Simulator/Quadcopter/Actuators ==
  Th1 [%] : Inport
  Th2 [%] : Inport  Port=2
  Th3 [%] : Inport  Port=3
  Th4 [%] : Inport  Port=4
  Constant : Constant  Value=0
  Demux2 : Demux
  ESC+Brushless1 : Subsystem
  ESC+Brushless2 : Subsystem
  ESC+Brushless3 : Subsystem
  ESC+Brushless4 : Subsystem
  Gain1 : Gain  Gain=K  Multiplication=Matrix(K*u)
  Math Function{,1..3} (4 alike) : Math  Operator=magnitude^2  SaturateOnIntegerOverflow=on
  Mux : Mux
  Mux1 : Mux  Inputs=3
  Mux2 : Mux  Inputs=3
  Transport Delay{,1..3} (4 alike) : TransportDelay  DelayTime=delay_mixer*tc
  Fprops : Outport
  Mprops : Outport  Port=2
  wires:
  Gain1/1 -> Demux2/1  "U"
  Th1 [%]/1 -> Transport Delay/1  "Throttle1 [%]"
  Th2 [%]/1 -> Transport Delay1/1  "Throttle2 [%]"
  Th4 [%]/1 -> Transport Delay3/1  "Throttle4 [%]"
  Th3 [%]/1 -> Transport Delay2/1  "Throttle3 [%]"
  ESC+Brushless1/1(Ω1 [rad/s]) -> Math Function/1
  ESC+Brushless2/1(Ω2 [rad/s]) -> Math Function1/1
  ESC+Brushless3/1(Ω3 [rad/s]) -> Math Function2/1
  ESC+Brushless4/1(Ω4 [rad/s]) -> Math Function3/1
  Mux/1 -> Gain1/1  "Ω^2"
  Math Function/1 -> Mux/1
  Math Function1/1 -> Mux/2
  Math Function2/1 -> Mux/3
  Math Function3/1 -> Mux/4
  Mux1/1 -> Mprops/1
  Demux2/2 -> Mux1/1
  Demux2/3 -> Mux1/2
  Demux2/4 -> Mux1/3
  Demux2/1 -> Mux2/3
  Constant/1 -> Mux2/2, Mux2/1
  Mux2/1 -> Fprops/1
  Transport Delay/1 -> ESC+Brushless1/1(Throttle1 [%])
  Transport Delay1/1 -> ESC+Brushless2/1(Throttle2 [%])
  Transport Delay3/1 -> ESC+Brushless4/1(Throttle4 [%])
  Transport Delay2/1 -> ESC+Brushless3/1(Throttle3 [%])

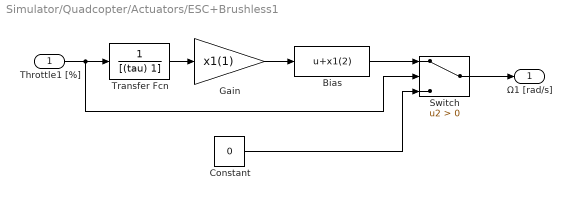
== system Simulator/Quadcopter/Actuators/ESC+Brushless1 ==
  Throttle1 [%] : Inport
  Bias : Bias  Bias=x1(2)
  Constant : Constant  Value=0
  Gain : Gain  Gain=x1(1)
  Switch : Switch  Criteria=u2 > Threshold
  Transfer Fcn : TransferFcn  Denominator=[(tau) 1]
  Ω1 [rad/s] : Outport
  wires:
  Gain/1 -> Bias/1
  Bias/1 -> Switch/1
  Constant/1 -> Switch/3
  Switch/1 -> Ω1 [rad/s]/1
  Throttle1 [%]/1 -> Transfer Fcn/1, Switch/2
  Transfer Fcn/1 -> Gain/1

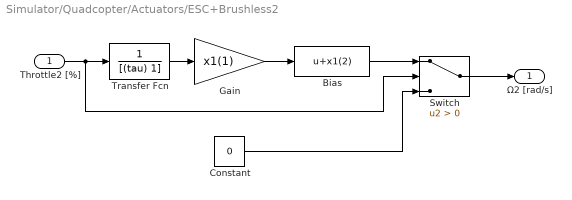
== system Simulator/Quadcopter/Actuators/ESC+Brushless2 ==
  Throttle2 [%] : Inport
  Bias : Bias  Bias=x1(2)
  Constant : Constant  Value=0
  Gain : Gain  Gain=x1(1)
  Switch : Switch  Criteria=u2 > Threshold
  Transfer Fcn : TransferFcn  Denominator=[(tau) 1]
  Ω2 [rad/s] : Outport
  wires:
  Switch/1 -> Ω2 [rad/s]/1
  Constant/1 -> Switch/3
  Bias/1 -> Switch/1
  Gain/1 -> Bias/1
  Throttle2 [%]/1 -> Transfer Fcn/1, Switch/2
  Transfer Fcn/1 -> Gain/1

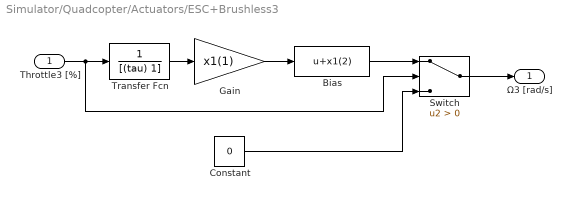
== system Simulator/Quadcopter/Actuators/ESC+Brushless3 ==
  Throttle3 [%] : Inport
  Bias : Bias  Bias=x1(2)
  Constant : Constant  Value=0
  Gain : Gain  Gain=x1(1)
  Switch : Switch  Criteria=u2 > Threshold
  Transfer Fcn : TransferFcn  Denominator=[(tau) 1]
  Ω3 [rad/s] : Outport
  wires:
  Gain/1 -> Bias/1
  Bias/1 -> Switch/1
  Constant/1 -> Switch/3
  Switch/1 -> Ω3 [rad/s]/1
  Throttle3 [%]/1 -> Transfer Fcn/1, Switch/2
  Transfer Fcn/1 -> Gain/1

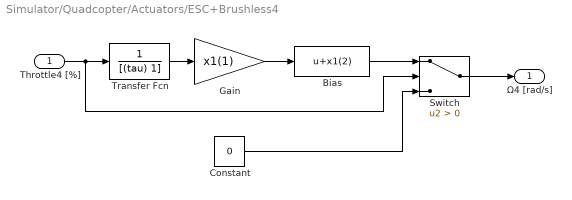
== system Simulator/Quadcopter/Actuators/ESC+Brushless4 ==
  Throttle4 [%] : Inport
  Bias : Bias  Bias=x1(2)
  Constant : Constant  Value=0
  Gain : Gain  Gain=x1(1)
  Switch : Switch  Criteria=u2 > Threshold
  Transfer Fcn : TransferFcn  Denominator=[(tau) 1]
  Ω4 [rad/s] : Outport
  wires:
  Switch/1 -> Ω4 [rad/s]/1
  Constant/1 -> Switch/3
  Bias/1 -> Switch/1
  Gain/1 -> Bias/1
  Throttle4 [%]/1 -> Transfer Fcn/1, Switch/2
  Transfer Fcn/1 -> Gain/1

== matlab function Simulator/Quadcopter/To body from Earth ==
  data: Alpha_e input; Earth input; body output
 function body = Tbe(Alpha_e, Earth)
%#codegen
phi = Alpha_e(1);
theta = Alpha_e(2);
psi = Alpha_e(3);

Sphi = sin(phi);
Cphi = cos(phi);
Stheta = sin(theta);
Ctheta = cos(theta);
Spsi = sin(psi);
Cpsi = cos(psi);

TBE = [        Ctheta*Cpsi               Ctheta*Spsi          -Stheta    ;
       Sphi*Stheta*Cpsi-Cphi*Spsi Sphi*Stheta*Spsi+Cphi*Cpsi Sphi*Ctheta ;
       Cphi*Stheta*Cpsi+Sphi*Spsi Cphi*Stheta*Spsi-Sphi*Cpsi Cphi*Ctheta];

body = TBE* Earth;

== matlab function Simulator/Quadcopter/To Earth from body ==
  data: Alpha_e input; Earth output; body input
 function Earth = Tbet(Alpha_e, body)
%#codegen
phi = Alpha_e(1);
theta = Alpha_e(2);
psi = Alpha_e(3);

Sphi = sin(phi);
Cphi = cos(phi);
Stheta = sin(theta);
Ctheta = cos(theta);
Spsi = sin(psi);
Cpsi = cos(psi);

TBE = [        Ctheta*Cpsi               Ctheta*Spsi          -Stheta    ;
       Sphi*Stheta*Cpsi-Cphi*Spsi Sphi*Stheta*Spsi+Cphi*Cpsi Sphi*Ctheta ;
       Cphi*Stheta*Cpsi+Sphi*Spsi Cphi*Stheta*Spsi-Sphi*Cpsi Cphi*Ctheta];
TEB = TBE';

Earth = TEB* body;

== matlab function Simulator/Quadcopter/To Earth from body_rates ==
  data: Alpha_e input; Rates_B input; Rates_E output
 function Rates_E = Einv(Alpha_e, Rates_B)
%#codegen
phi = Alpha_e(1);
theta = Alpha_e(2);

Sphi = sin(phi);
Cphi = cos(phi);
Ctheta = cos(theta);
Ttheta = tan(theta);

Einv = [1   Sphi*Ttheta    Cphi*Ttheta ;
        0       Cphi          -Sphi    ;
        0   Sphi/Ctheta    Cphi/Ctheta];

Rates_E = Einv* Rates_B;

== matlab function Simulator/Controllers/Attitude Controller/To body from Earth_rates ==
  data: Alpha_e input; Rates_B output; Rates_E input
 function Rates_B = E(Alpha_e, Rates_E)
%#codegen
phi = Alpha_e(1);
theta = Alpha_e(2);

Sphi = sin(phi);
Cphi = cos(phi);
Stheta = sin(theta);
Ctheta = cos(theta);

E = [1      0        -Stheta   ;
     0     Cphi    Sphi*Ctheta ;
     0    -Sphi    Cphi*Ctheta];

Rates_B = E* Rates_E;

== matlab function Simulator/Controllers/Position Controller/To Earth from body ==
  data: Head input; dXY output; dNE input
 function dXY = T(Head, dNE)
%#codegen
psi = Head;

Spsi = sin(psi);
Cpsi = cos(psi);

T = [ Cpsi Spsi ;
     -Spsi Cpsi];

dXY = T * dNE;
